simulink model "ABS_simulink"  (R2015b)
settings: Solver=ode1  StartTime=0.0  StopTime=Inf  FixedStep=0.001  RelTol=1e-3
PostLoadFcn:
  | , if any(exist('dsrtsu_mdlpostloadfcn', 'file') == [2, 3, 6]), try dsrtsu_mdlpostloadfcn('Execute', bdroot); catch fprintf('Error in PostLoadFcn (dsrtsu_mdlpostloadfcn) for model "%s":\n %s\n', bdroot, lasterr); end, end,
values from neighbouring files (symbols this model uses):
  A = [-a/v  1/v ... (first row only)    [ABS_mpcdesign.m]    (also in mpc_ssMatrix.m = [0.299843671875         0)
  actuatorDelay = 0.005    [Fahrzeug_Parameter.m]
  actuatorPole = 70    [Fahrzeug_Parameter.m]
  actuatorSat = 4000    [Fahrzeug_Parameter.m]
  B = [0 ... (first row only)    [ABS_mpcdesign.m]    (also in mpc_ssMatrix.m = [0.010667   0.010667)
  C = [Fz*K_mu*R  J]    [ABS_mpcdesign.m]    (also in mpc_ssMatrix.m = [1           0)
  D = [0]    [ABS_mpcdesign.m]    (also in mpc_ssMatrix.m = zeros(2,2))
  g = 9.81    [ABS_mpcdesign.m]    (also in ABS_mpcfahrzeugpara.m; Fahrzeug_Parameter.m)
  J = 1    [ABS_mpcdesign.m]    (also in ABS_mpcfahrzeugpara.m)
  m = 2    [ABS_mpcdesign.m]    (also in ABS_mpcfahrzeugpara.m = 450; Fahrzeug_Parameter.m = 450; mpc_ssMatrix.m; mpc_withConstrains.m)
  roadCoeffs = [1.28 23.99 0.52]    [Fahrzeug_Parameter.m]
  Rr = 0.32    [Fahrzeug_Parameter.m]
  Td = 1500    [ABS_mpcdesign.m]    (also in ABS_mpcfahrzeugpara.m; Fahrzeug_Parameter.m)
  v0 = 50    [Fahrzeug_Parameter.m]
libraries: simulink x1, mpclib x1
settings Model: DSRTSU_INTERNAL_RTI_VER=470  DSRTSU_INTERNAL_RTI_TYPE=rti1401  DSRTSU_INTERNAL_RTIFPGA=60  Creator=MSI  LastModifiedBy=MSI
settings OptimizationCC: BlockReduction=off  OptimizeBlockIOStorage=off  BufferReuse=off  GlobalBufferReuse=off  ExpressionFolding=off  LocalBlockOutputs=off
settings HardwareCC: ProdBitPerPointer=32  ProdLargestAtomicInteger=Integer  ProdEndianess=BigEndian  ProdWordSize=32  ProdHWDeviceType=Custom Processor->Custom  TargetIntDivRoundTo=Zero  TargetEndianess=BigEndian  TargetHWDeviceType=Custom Processor->Custom
settings RTWCC: SystemTargetFile=rti1401.tlc  MakeCommand=make_rti  TemplateMakefile=rti1401.tmf  Description=dSPACE DS1401 Hardware Platform
settings STFCustomTargetCC: ParMdlRefBuildCompliant=on  ConcurrentExecutionCompliant=off  GeneratePreprocessorConditionals=Use local settings  MatFileLogging=on  CPPClassGenCompliant=off  SystemTargetFile=rti1401.tlc
settings GRTTargetCC: CompOptLevelCompliant=off  ConcurrentExecutionCompliant=off  CombineOutputUpdateFcns=off  CPPClassGenCompliant=off  GRTInterface=on  UseToolchainInfoCompliant=off  ExtModeMexFile=noextcomm

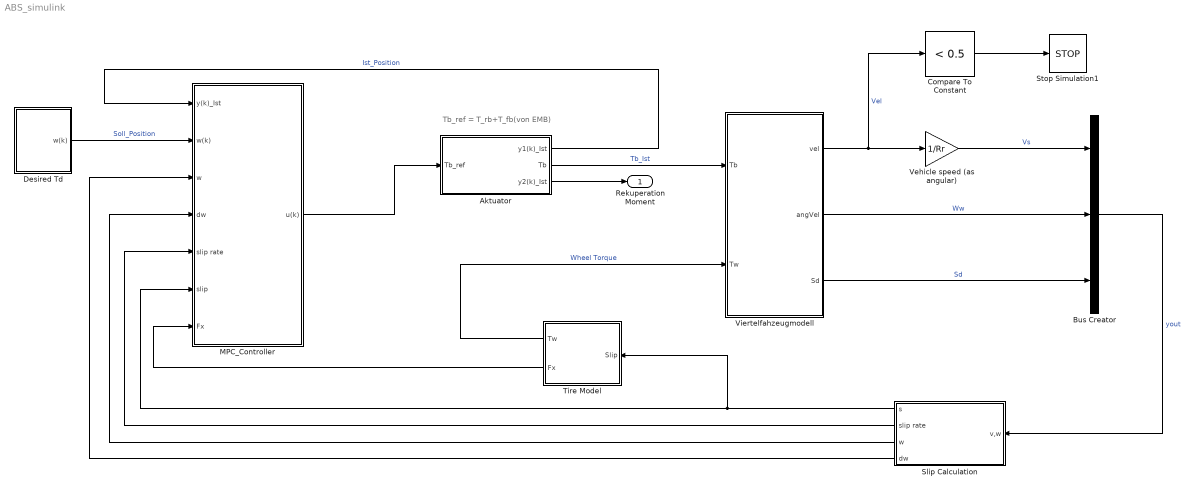
== system ABS_simulink ==
  note: Tb_ref = T_rb+T_fb(von EMB)
  Aktuator : Subsystem  TreatAsAtomicUnit=on
      settings: MinAlgLoopOccurrences=on
  Bus Creator : BusCreator  Inputs=3
  Compare To Constant : simulink/Logic and Bit Operations/Compare To Constant  relop=<  const=0.5  OutDataTypeStr=boolean
  Desired Td : Subsystem
  MPC_Controller : Subsystem
  Slip Calculation : Subsystem
  Stop Simulation1 : Stop
  Tire Model : Subsystem
  "Vehicle speed (as angular)  " : Gain  Gain=1/Rr
  Viertelfahzeugmodell : Subsystem
  Rekuperation Moment : Outport
  wires:
  Tire Model/2(Fx) -> MPC_Controller/7(Fx)
  Tire Model/1(Tw) -> Viertelfahzeugmodell/2(Tw)  "Wheel Torque"
  "Vehicle speed (as angular)  "/1 -> Bus Creator/1  "Vs"
  Viertelfahzeugmodell/1(vel) -> "Vehicle speed (as angular)  "/1, Compare To Constant/1  "Vel"
  Viertelfahzeugmodell/2(angVel) -> Bus Creator/2  "Ww"
  Compare To Constant/1 -> Stop Simulation1/1
  Bus Creator/1 -> Slip Calculation/1(v,w)  "yout"
  Viertelfahzeugmodell/3(Sd) -> Bus Creator/3  "Sd"
  Aktuator/2(Tb) -> Viertelfahzeugmodell/1(Tb)  "Tb_Ist"
  MPC_Controller/1(u(k)) -> Aktuator/1(Tb_ref)
  Slip Calculation/1(s) -> Tire Model/1(Slip), MPC_Controller/6(slip)
  Slip Calculation/3(w) -> MPC_Controller/4(dw)
  Desired Td/1(w(k)) -> MPC_Controller/2(w(k))  "Soll_Position"
  Aktuator/1(y1(k)_Ist) -> MPC_Controller/1(y(k)_Ist)  "Ist_Position"
  Slip Calculation/4(dw) -> MPC_Controller/3(w)
  Slip Calculation/2(slip rate) -> MPC_Controller/5(slip rate)
  Aktuator/3(y2(k)_Ist) -> Rekuperation Moment/1

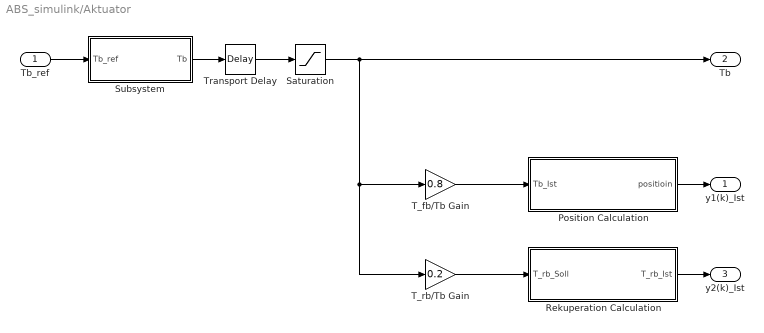
== system ABS_simulink/Aktuator ==
  Tb_ref : Inport
  Position Calculation : Subsystem
  Rekuperation Calculation : Subsystem
  Saturation : Saturate  UpperLimit=actuatorSat  LowerLimit=0
  Subsystem : Subsystem
  T_fb/Tb Gain : Gain  Gain=0.8
  T_rb/Tb Gain : Gain  Gain=0.2
  Transport Delay : TransportDelay  DelayTime=actuatorDelay  BufferSize=10240
  y1(k)_Ist : Outport
  Tb : Outport  Port=2
  y2(k)_Ist : Outport  Port=3
  wires:
  Transport Delay/1 -> Saturation/1
  Tb_ref/1 -> Subsystem/1(Tb_ref)
  Subsystem/1(Tb) -> Transport Delay/1
  Saturation/1 -> T_rb/Tb Gain/1, T_fb/Tb Gain/1, Tb/1
  Position Calculation/1(" positioin") -> y1(k)_Ist/1
  T_fb/Tb Gain/1 -> Position Calculation/1(Tb_Ist)
  T_rb/Tb Gain/1 -> Rekuperation Calculation/1(T_rb_Soll)
  Rekuperation Calculation/1(" T_rb_Ist") -> y2(k)_Ist/1

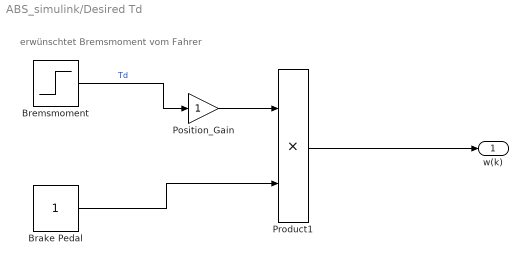
== system ABS_simulink/Desired Td ==
  note: erwünschtet Bremsmoment vom Fahrer
  Brake Pedal : Constant  OutMin=[0]  OutMax=[1]
  Bremsmoment : Step  After=Td  SampleTime=0
  Position_Gain : Gain
  Product1 : Product  SaturateOnIntegerOverflow=on  OutDataTypeStr=Inherit: Same as first input
  w(k) : Outport
  wires:
  Product1/1 -> w(k)/1
  Bremsmoment/1 -> Position_Gain/1  "Td"
  Brake Pedal/1 -> Product1/2
  Position_Gain/1 -> Product1/1

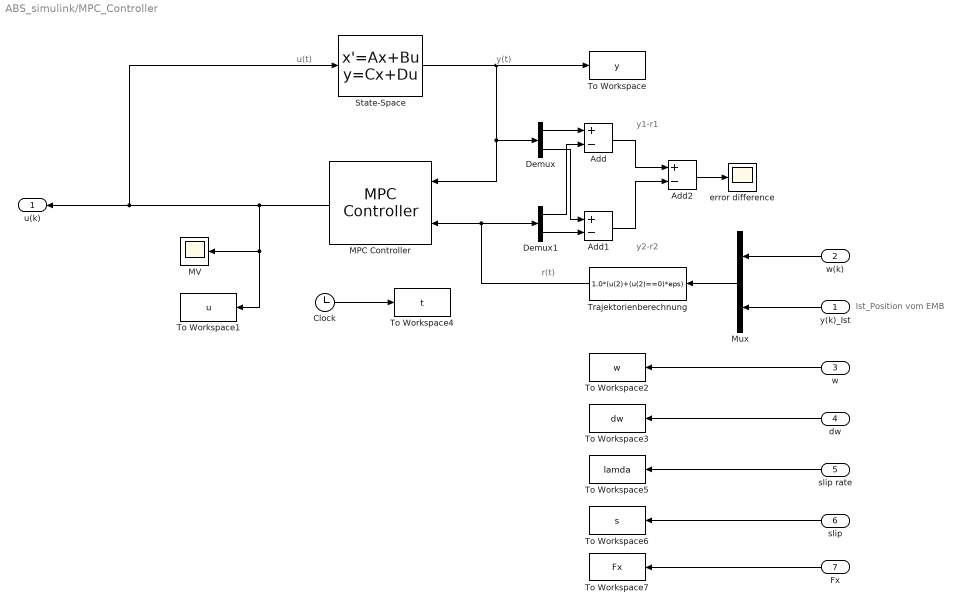
== system ABS_simulink/MPC_Controller ==
  note: y2-r2
  note: y1-r1
  note: r(t)
  note: y(t)
  note: u(t)
  note: Ist_Position vom EMB
  y(k)_Ist : Inport
  w(k) : Inport  Port=2
  w : Inport  Port=3
  dw : Inport  Port=4
  slip rate : Inport  Port=5
  slip : Inport  Port=6
  Fx : Inport  Port=7
  Add : Sum  Inputs=+-
  Add1 : Sum  Inputs=+-
  Add2 : Sum  Inputs=+-
  Clock : Clock
  Demux : Demux  Outputs=2
  Demux1 : Demux  Outputs=2
  MPC Controller : mpclib/MPC Controller  mpcobj=mpcobj  x0=[]  is_multiple=0  enable_value=0  return_u0=off  ref_from_ws=off  ref_signal_name=[]  ref_preview=on  md_from_ws=off  md_signal_name=[]  md_preview=on  from_project=off  project_file=MPCtask.mat  md_inport=off  mv_inport=off  cost_outport=off  return_sequence=off  return_qpstatus=off  return_state=off  state_inport=off  lims_inport=off  ywt_inport=off  is_designfromscratch=0  uwt_inport=off  duwt_inport=off  rhoeps_inport=off  uref_inport=off  n_ts=0.1  n_mv=2  n_md=0  n_ud=0  n_mo=2  n_uo=0  BlockDataType=double  SampleTimeInherited=off  switch_inport=off
  MV : Scope
  Mux : Mux  Inputs=2
  State-Space : StateSpace  A=A  B=B  C=C  D=D  X0=[0 0 0 0 0 0 0]'
  To Workspace : ToWorkspace  VariableName=y  SampleTime=-1
      settings: MaxDataPoints=Inf
  To Workspace1 : ToWorkspace  VariableName=u  SampleTime=-1
      settings: MaxDataPoints=Inf
  To Workspace2 : ToWorkspace  VariableName=w  SampleTime=-1
      settings: MaxDataPoints=Inf
  To Workspace3 : ToWorkspace  VariableName=dw  SampleTime=-1
      settings: MaxDataPoints=Inf
  To Workspace4 : ToWorkspace  VariableName=t  SampleTime=-1
      settings: MaxDataPoints=Inf
  To Workspace5 : ToWorkspace  VariableName=lamda  SampleTime=-1
      settings: MaxDataPoints=Inf
  To Workspace6 : ToWorkspace  VariableName=s  SampleTime=-1
      settings: MaxDataPoints=Inf
  To Workspace7 : ToWorkspace  VariableName=Fx  SampleTime=-1
      settings: MaxDataPoints=Inf
  Trajektorienberechnung : Fcn  Expr=1.0*(u(2)+(u(2)==0)*eps)
  error difference : Scope
  u(k) : Outport
  wires:
  MPC Controller/1 -> u(k)/1, State-Space/1, To Workspace1/1, MV/1
  y(k)_Ist/1 -> Mux/2
  w(k)/1 -> Mux/1
  Add2/1 -> error difference/1
  Add1/1 -> Add2/2
  Add/1 -> Add2/1
  Demux1/2 -> Add1/2
  Demux/2 -> Add1/1
  Demux1/1 -> Add/2
  Demux/1 -> Add/1
  Clock/1 -> To Workspace4/1
  State-Space/1 -> Demux/1, MPC Controller/1, To Workspace/1
  Mux/1 -> Trajektorienberechnung/1
  Trajektorienberechnung/1 -> Demux1/1, MPC Controller/2
  w/1 -> To Workspace2/1
  dw/1 -> To Workspace3/1
  slip rate/1 -> To Workspace5/1
  slip/1 -> To Workspace6/1
  Fx/1 -> To Workspace7/1

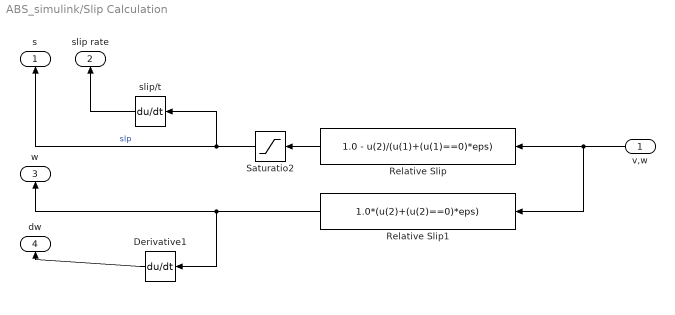
== system ABS_simulink/Slip Calculation ==
  v,w : Inport
  Derivative1 : Derivative
  Relative Slip : Fcn  Expr=1.0 - u(2)/(u(1)+(u(1)==0)*eps)
  Relative Slip1 : Fcn  Expr=1.0*(u(2)+(u(2)==0)*eps)
  Saturatio2 : Saturate  UpperLimit=1  LowerLimit=0
  slip/t : Derivative
  s : Outport
  slip rate : Outport  Port=2
  w : Outport  Port=3
  dw : Outport  Port=4
  wires:
  Relative Slip/1 -> Saturatio2/1
  v,w/1 -> Relative Slip1/1, Relative Slip/1
  Saturatio2/1 -> s/1, slip/t/1  "slp"
  Relative Slip1/1 -> Derivative1/1, w/1
  slip/t/1 -> slip rate/1
  Derivative1/1 -> dw/1

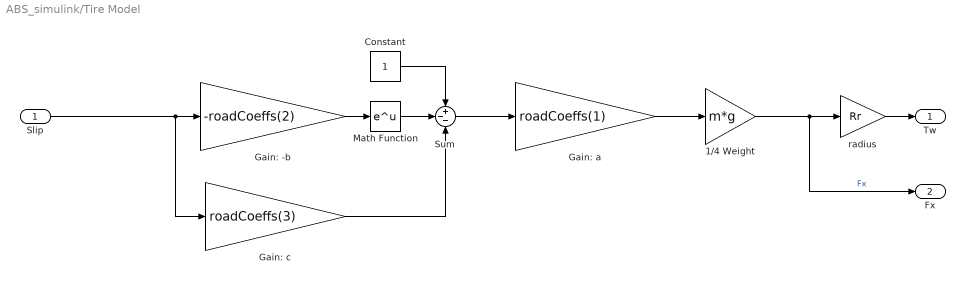
== system ABS_simulink/Tire Model ==
  Slip : Inport
  1/4 Weight : Gain  Gain=m*g
  Constant : Constant
  Gain: -b : Gain  Gain=-roadCoeffs(2)  SaturateOnIntegerOverflow=on  OutDataTypeStr=Inherit: Same as input  ParamDataTypeStr=Inherit: Same as input
  Gain: a : Gain  Gain=roadCoeffs(1)  SaturateOnIntegerOverflow=on  OutDataTypeStr=Inherit: Same as input  ParamDataTypeStr=Inherit: Same as input
  Gain: c : Gain  Gain=roadCoeffs(3)  SaturateOnIntegerOverflow=on  OutDataTypeStr=Inherit: Same as input  ParamDataTypeStr=Inherit: Same as input
  Math Function : Math  SaturateOnIntegerOverflow=on
  Sum : Sum  Inputs=+--
  radius : Gain  Gain=Rr  SaturateOnIntegerOverflow=on  OutDataTypeStr=Inherit: Same as input  ParamDataTypeStr=Inherit: Same as input
  Tw : Outport
  Fx : Outport  Port=2
  wires:
  radius/1 -> Tw/1
  Gain: a/1 -> 1/4 Weight/1
  1/4 Weight/1 -> Fx/1, radius/1  "Fx"
  Slip/1 -> Gain: -b/1, Gain: c/1
  Gain: -b/1 -> Math Function/1
  Math Function/1 -> Sum/2
  Constant/1 -> Sum/1
  Gain: c/1 -> Sum/3
  Sum/1 -> Gain: a/1

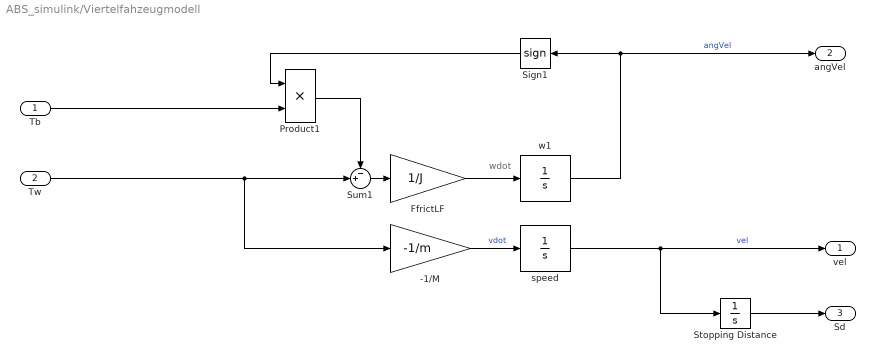
== system ABS_simulink/Viertelfahzeugmodell ==
  note: wdot
  Tb : Inport
  Tw : Inport  Port=2
  -1/M : Gain  Gain=-1/m  SaturateOnIntegerOverflow=on  OutDataTypeStr=Inherit: Same as input  ParamDataTypeStr=Inherit: Same as input
  FfrictLF : Gain  Gain=1/J  SaturateOnIntegerOverflow=on  OutDataTypeStr=Inherit: Same as input  ParamDataTypeStr=Inherit: Same as input
  Product1 : Product  SaturateOnIntegerOverflow=on  OutDataTypeStr=Inherit: Same as first input
  Sign1 : Signum
  Stopping Distance : Integrator
  Sum1 : Sum  Inputs=-+|
  speed : Integrator  InitialCondition=v0  LimitOutput=on  UpperSaturationLimit=1000  LowerSaturationLimit=0
  w1 : Integrator  LimitOutput=on  UpperSaturationLimit=1500  LowerSaturationLimit=0
  vel : Outport
  angVel : Outport  Port=2
  Sd : Outport  Port=3
  wires:
  Stopping Distance/1 -> Sd/1
  Tb/1 -> Product1/2
  Product1/1 -> Sum1/1
  Tw/1 -> -1/M/1, Sum1/2
  Sum1/1 -> FfrictLF/1
  speed/1 -> vel/1, Stopping Distance/1  "vel"
  w1/1 -> angVel/1, Sign1/1  "angVel"
  Sign1/1 -> Product1/1
  FfrictLF/1 -> w1/1
  -1/M/1 -> speed/1  "vdot"

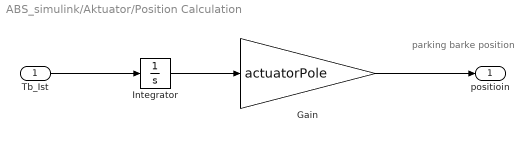
== system ABS_simulink/Aktuator/Position Calculation ==
  note: parking barke position
  Tb_Ist : Inport
  Gain : Gain  Gain=actuatorPole
  Integrator : Integrator
  " positioin" : Outport
  wires:
  Gain/1 -> " positioin"/1
  Tb_Ist/1 -> Integrator/1
  Integrator/1 -> Gain/1

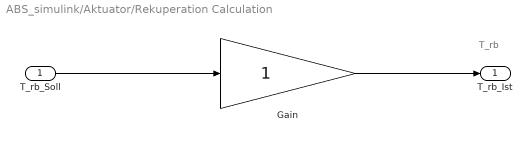
== system ABS_simulink/Aktuator/Rekuperation Calculation ==
  note: T_rb
  T_rb_Soll : Inport
  Gain : Gain
  " T_rb_Ist" : Outport
  wires:
  Gain/1 -> " T_rb_Ist"/1
  T_rb_Soll/1 -> Gain/1

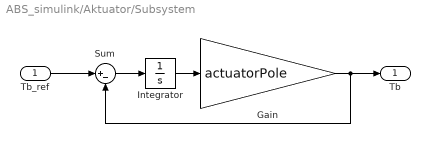
== system ABS_simulink/Aktuator/Subsystem ==
  Tb_ref : Inport
  Gain : Gain  Gain=actuatorPole
  Integrator : Integrator
  Sum : Sum  Inputs=|+-
  Tb : Outport
  wires:
  Integrator/1 -> Gain/1
  Sum/1 -> Integrator/1
  Tb_ref/1 -> Sum/1
  Gain/1 -> Sum/2, Tb/1
